simulink model "Sub1"  (R2024a)
settings: Solver=FixedStepDiscrete  StartTime=0.0  StopTime=1  FixedStep=7.5e-05  RelTol=1e-3  EnableMultiTasking=on
undefined symbols (not defined in the file or in its folder): D1, D11, Delta
libraries: spsSeriesRLCBranchLib x41, spsLoadFlowBusLib x29, spsDistributedParametersLineLib x19, spsThreePhaseSeriesRLCLoadLib x15, spsThreePhaseTransformerTwoWindingsLib x13, spsThreePhaseParallelRLCLoadLib x11, spsThreePhaseVIMeasurementLib x11, spsSynchronousMachinepuStandardLib x7, spsExcitationSystemLib x7, spsHydraulicTurbineandGovernorLib x7, spsGenericPowerSystemStabilizerLib x7, spsMultiBandPowerSystemStabilizerLib x7
(part 3 of 5)

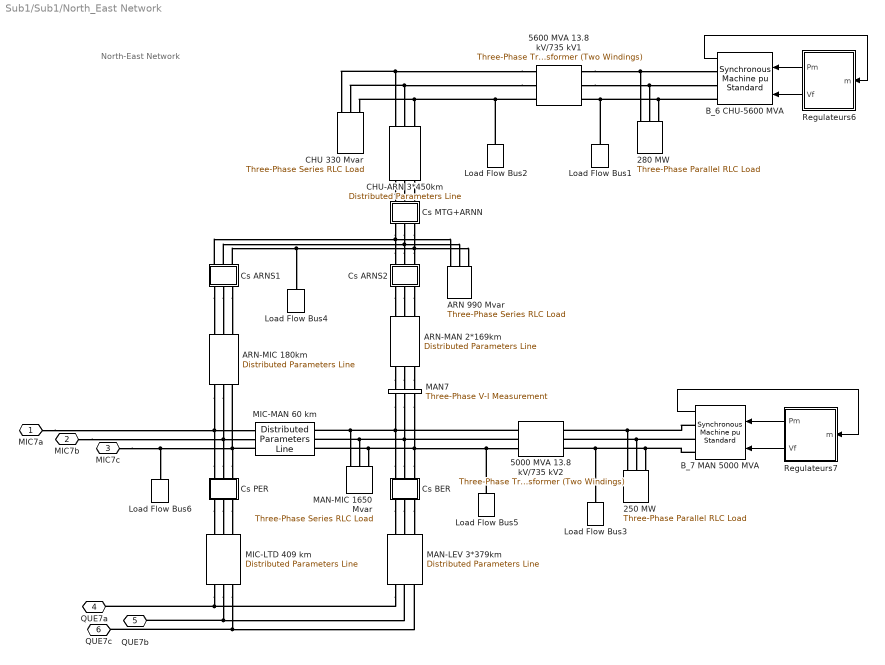
== system Sub1/Sub1/North_East Network ==
  note: North-East Network
  250 MW : spsThreePhaseParallelRLCLoadLib/Three-Phase Parallel RLC Load  LConnTagsString=A|B|C  Configuration=Y (grounded)  NominalVoltage=(13800)*1  Vabc=[1e3 1e3 1e3]  Vabcp=[1e3 1e3 1e3]  NominalFrequency=60  UnbalancedPower=off  ActivePower=250000000  InductivePower=0  CapacitivePower=0  Pabc=[10e3 9e3 11e3]  QLabc=[100 90 110]  QCabc=[100 90 110]  Pabcp=[10e3 9e3 11e3]  QLabcp=[100 90 110]  QCabcp=[100 90 110]  Measurements=None  LoadType=constant PQ
  280 MW : spsThreePhaseParallelRLCLoadLib/Three-Phase Parallel RLC Load  LConnTagsString=A|B|C  Configuration=Y (grounded)  NominalVoltage=(13800)*1  Vabc=[1e3 1e3 1e3]  Vabcp=[1e3 1e3 1e3]  NominalFrequency=60  UnbalancedPower=off  ActivePower=280000000  InductivePower=0  CapacitivePower=0  Pabc=[10e3 9e3 11e3]  QLabc=[100 90 110]  QCabc=[100 90 110]  Pabcp=[10e3 9e3 11e3]  QLabcp=[100 90 110]  QCabcp=[100 90 110]  Measurements=None  LoadType=constant PQ
  5000 MVA 13.8 kV/735 kV2 : spsThreePhaseTransformerTwoWindingsLib/Three-Phase Transformer (Two Windings)  Winding1Connection=Delta (D1)  Winding2Connection=Yg  CoreType=Three single-phase transformers  SetSaturation=off  Hysteresis=off  DataFile='basic_model'  SetInitialFlux=off  Measurements=None  UNITS=pu  NominalPower=[ 5000e6 60 ]  Winding1="[ 13.8e3 0.002  0.0]"  Winding2=[ 735e3 0.002 0.12]  Rm=500  Lm=500  L0=0.5  Saturation="[ 0,0  ;  0.005,1.2  ;  1.0,1.4 ]"  InitialFluxes=[ 0.8 , -0.8 , 0.7 ]  BreakLoop=off  DiscreteSolver=Trapezoidal iterative  DataType=off  TransfoNumber=0
  5600 MVA 13.8 kV/735 kV1 : spsThreePhaseTransformerTwoWindingsLib/Three-Phase Transformer (Two Windings)  Winding1Connection=Delta (D1)  Winding2Connection=Yg  CoreType=Three single-phase transformers  SetSaturation=off  Hysteresis=off  DataFile='basic_model'  SetInitialFlux=off  Measurements=None  UNITS=pu  NominalPower=[ 5600e6 60 ]  Winding1="[ 13.8e3 0.002  0.0]"  Winding2=[ 735e3 0.002 0.12]  Rm=500  Lm=500  L0=0.5  Saturation="[ 0,0  ;  0.005,1.2  ;  1.0,1.4 ]"  InitialFluxes=[ 0.8 , -0.8 , 0.7 ]  BreakLoop=off  DiscreteSolver=Trapezoidal iterative  DataType=off  TransfoNumber=0
  ARN 990 Mvar : spsThreePhaseSeriesRLCLoadLib/Three-Phase Series RLC Load  LConnTagsString=A|B|C  Configuration=Y (grounded)  NominalVoltage=735e3  Vabc=[1e3 1e3 1e3]  Vabcp=[1e3 1e3 1e3]  NominalFrequency=60  UnbalancedPower=off  ActivePower=3300000  InductivePower=990e6  CapacitivePower=0  Pabc=[10e3 9e3 11e3]  QLabc=[100 90 110]  QCabc=[100 90 110]  Pabcp=[10e3 9e3 11e3]  QLabcp=[100 90 110]  QCabcp=[100 90 110]  Measurements=None  LoadType=constant Z
  ARN-MAN 2*169km : spsDistributedParametersLineLib/Distributed Parameters Line  Phases=3  Length=169  Frequency=60  Resistance="[0.01273  0.3864]/2"  Inductance="[0.9337e-3  4.1264e-3]/2"  Capacitance=[12.74e-9 7.751e-9]*2  x1=[-0.000975 1.40296657323216e-09 347873.977312495 -681165.145140608;-0.0009 1.33832794722541e-09 366991.883229389 -671058.367401907;-0.000825 1.27261948233475e-09 385816.421449993 -660415.155871841;-0.00075 1.20589370490164e-09 404332.543926479 -649244.018570862;-0.000675 1.13820395449163e-09 422525.449153847 -637553.885535204;-0.0006 1.0696043412555e-09 440380.594002016 -625354.101678351;-0.000525 1.00014970267447e-09 457883.70534139 -612654.419320855;-0.00045 9.29895559723926e-10 475020.791452569 -599464.990394481;-0.000375 8.58898072490815e-10 491778.153211123 -585796.358326908;-0.0003 7.87213995280137e-10 508142.395038458 -571659.449613472;-0.000225 7.1490063124641e-10 524100.435610038 -557065.565082699;-0.00015 6.4201578658641e-10 539639.518312398 -542026.370862587;-7.5e-05 5.68617724329785e-10 554747.22144058 -526553.88905489]  x2=[-0.000975 1.15383562490741e-09 232985.418240247 -689450.364518719;-0.0009 1.12361481292558e-09 252383.458947585 -682588.200671908;-0.000825 1.09249580045418e-09 271579.748179437 -675180.38626143;-0.00075 1.06050346355564e-09 290558.940715904 -667232.84298078;-0.000675 1.02766337641458e-09 309305.864880863 -658751.923974457;-0.0006 9.940017908942e-10 327805.534669975 -649744.408759351;-0.000525 9.59545615550911e-10 346043.161730265 -640217.497805305;-0.00045 9.24322394124092e-10 364004.167181706 -630178.80677917;-0.000375 8.88360283518016e-10 381674.193271352 -619636.360456955;-0.0003 8.51688031293665e-10 399039.114850707 -608598.586308945;-0.000225 8.14334952688361e-10 416085.050667155 -597074.30776291;-0.00015 7.76330907181621e-10 432798.374460414 -585072.737150793;-7.5e-05 7.37706274625941e-10 449165.725855166 -572603.46834451]  x3=[-0.000975 -7.73577503889558e-12 1583.75858462524 -1421.24992657483;-0.0009 -7.93874680673473e-12 1623.30400424471 -1375.90902523544;-0.000825 -8.13537246184348e-12 1661.55177948056 -1329.46824327338;-0.00075 -8.3254948246816e-12 1698.4713356465 -1281.96470473921;-0.000675 -8.50896191434122e-12 1734.0331598142 -1233.43638323478;-0.0006 -8.68562707003799e-12 1768.20882440554 -1183.9220715578;-0.000525 -8.85534906834953e-12 1800.97100991715 -1133.46135069143;-0.00045 -9.01799223610721e-12 1832.29352675922 -1082.09455816387;-0.000375 -9.17342655885125e-12 1862.15133619103 -1029.8627558031;-0.0003 -9.32152778476228e-12 1890.52057033656 -976.807696912781;-0.000225 -9.46217752398633e-12 1917.37855126409 -922.971792895205;-0.00015 -9.59526334327388e-12 1942.70380911462 -868.398079348331;-7.5e-05 -9.72067885585727e-12 1966.47609926451 -813.130181663762]  x4=[-0.000975 1.24888211846857e-11 1569.30174481143 -9115.59279820371;-0.0009 1.24221857541019e-11 1826.37892658961 -9067.58416140515;-0.000825 1.23456202182921e-11 2081.99612899841 -9012.32703656664;-0.00075 1.22591857825741e-11 2335.94901555729 -8949.86559538834;-0.000675 1.21629515413134e-11 2588.03458021436 -8880.24976859062;-0.0006 1.20569944226899e-11 2838.05130962626 -8803.53520600026;-0.000525 1.19413991272031e-11 3085.79934424489 -8719.78323206483;-0.00045 1.18162580599636e-11 3331.08063808204 -8629.06079683085;-0.000375 1.16816712568257e-11 3573.69911702436 -8531.44042242494;-0.0003 1.15377463044207e-11 3813.46083557195 -8427.00014508076;-0.000225 1.13845982541534e-11 4050.17413187549 -8315.82345275802;-0.00015 1.12223495302319e-11 4283.64978094776 -8197.99921840352;-7.5e-05 1.10511298318037e-11 4513.70114592717 -8073.62162890742]  x5=0.000955765248222805  V1=ones(3,3)  V2=ones(3,3)  I1=ones(3,3)  I2=ones(3,3)  nHarmo=1  Measurements=None  Decoupling=on  VsMag0=[624500.542746134 624501.904306159 624500.043261812]  VrMag0=[594207.380493459 594208.101305642 594207.286862208]  VsAngle0=[18.1135948354262 -101.886530201493 138.113424134256]  VrAngle0=[9.73160889880125 -110.268441654035 129.731523430557]  IsMag0=[1744.35611857435 1744.39210598318 1744.37536737656]  IrMag0=[7582.44376493559 7582.43378992651 7582.40838116995]  IsAngle0=[39.1559168024892 -80.8440356055455 159.154916919477]  IrAngle0=[0.828149284036614 -119.172115933988 120.828081951992]
      settings: AttributesFormatString=\n  LibrarySourceBlock=sps_lib/Power Grid Elements/Distributed Parameters Line
  ARN-MIC 180km : spsDistributedParametersLineLib/Distributed Parameters Line  Phases=3  Length=180  Frequency=60  Resistance="[0.01273  0.3864]"  Inductance="[0.9337e-3  4.1264e-3]"  Capacitance=[12.74e-9 7.751e-9]  x1=[-0.00105 1.26488530745679e-09 336203.730988093 -674396.627297763;-0.000975 1.2044174612995e-09 355134.952563311 -664622.476598035;-0.0009 1.14298682225185e-09 373782.284691197 -654317.03685958;-0.000825 1.08064249702677e-09 392130.820979761 -643488.546093246;-0.00075 1.01743432272396e-09 410165.893889837 -632145.660428869;-0.000675 9.53412826990829e-10 427873.086460087 -620297.447195699;-0.0006 8.88629187631506e-10 445238.243831697 -607953.377674109;-0.000525 8.23135191696074e-10 462247.484563562 -595123.319524406;-0.00045 7.5698319408279e-10 478887.211728891 -581817.528898766;-0.000375 6.90226075686387e-10 495144.123784384 -568046.642242632;-0.0003 6.22917201125894e-10 511005.225203283 -553821.667792094;-0.000225 5.55110376085774e-10 526457.836863796 -539153.976774079;-0.00015 4.86859804304484e-10 541489.606184596 -524055.294316363;-7.5e-05 4.18220044244838e-10 556088.51699928 -508537.690074686]  x2=[-0.00105 4.67164063168132e-09 192165.578486796 -719334.039084833;-0.000975 4.62687418731474e-09 212424.764832653 -713613.931123211;-0.0009 4.57840909051637e-09 232514.142071711 -707323.371103708;-0.000825 4.52628408354304e-09 252417.651063182 -700467.387603755;-0.00075 4.47054083432781e-09 272119.381246513 -693051.461191662;-0.000675 4.41122390317118e-09 291603.583360041 -685081.520045535;-0.0006 4.34838070712034e-09 310854.682030716 -676563.935214383;-0.000525 4.28206148206469e-09 329857.288224812 -667505.515525196;-0.00045 4.21231924257801e-09 348596.211549686 -657913.502140075;-0.000375 4.13920973953947e-09 367056.472396749 -647795.562767757;-0.0003 4.06279141556716e-09 385223.31391593 -637159.785534167;-0.000225 3.98312535830005e-09 403082.213812081 -626014.672516893;-0.00015 3.90027525156537e-09 420618.895953875 -614369.132948754;-7.5e-05 3.8143073244708e-09 437819.341785928 -602232.476095899]  x3=[-0.00105 2.81387396252104e-12 149.00166074934 -364.54093553834;-0.000975 3.09923380082505e-12 159.247423691766 -360.183291872447;-0.0009 3.38211615904855e-12 169.36588668026 -355.53772319402;-0.000825 3.66229490536262e-12 179.348961170327 -350.607943099582;-0.00075 3.93954606916433e-12 189.188666844966 -345.397892379912;-0.000675 4.21364802011543e-12 198.877137994012 -339.911735869838;-0.0006 4.48438164531022e-12 208.406629801869 -334.153859118933;-0.000525 4.7515305244311e-12 217.76952453859 -328.128864885774;-0.00045 5.0148811027516e-12 226.95833764938 -321.841569458566;-0.000375 5.27422286184881e-12 235.965723737633 -315.296998805074;-0.0003 5.52934848788858e-12 244.784482436726 -308.500384554942;-0.000225 5.780054037349e-12 253.407564165887 -301.457159817612;-0.00015 6.02613910004975e-12 261.82807576552 -294.172954839173;-7.5e-05 6.26740695935695e-12 270.03928600749 -286.653592501632]  x4=[-0.00105 5.46621407801285e-12 1187.65933351911 -4979.4651542706;-0.000975 5.11013850401405e-12 1327.95758028632 -4943.89904376687;-0.0009 4.74997796348289e-12 1467.19427808228 -4904.38085601174;-0.000825 4.38602036324481e-12 1605.25812322116 -4860.94218123987;-0.00075 4.01855664543673e-12 1742.03874957762 -4813.61774366322;-0.000675 3.64788055493226e-12 1877.42681681175 -4762.44537371311;-0.0006 3.27428840452662e-12 2011.31409777411 -4707.46597779911;-0.000525 2.89807883806869e-12 2143.59356502085 -4648.7235056091;-0.00045 2.5195525917297e-12 2274.1594763698 -4586.26491497656;-0.000375 2.13901225359934e-12 2402.90745942914 -4520.1401343432;-0.0003 1.75676202180143e-12 2529.73459503113 -4450.40202284691;-0.000225 1.37310746132265e-12 2654.53949950409 -4377.10632806698;-0.00015 9.88355259748543e-13 2777.22240571696 -4300.31164146037;-7.5e-05 6.02812982102133e-13 2897.68524283163 -4220.07935152456]  x5=0.00101797482059234  V1=ones(3,3)  V2=ones(3,3)  I1=ones(3,3)  I2=ones(3,3)  nHarmo=1  Measurements=None  Decoupling=on  VsMag0=[615273.936100305 615275.237958967 615273.425866952]  VrMag0=[607930.231676096 607930.976808471 607930.152146782]  VsAngle0=[19.177410374195 -100.822714483797 139.17724295489]  VrAngle0=[7.63692875075284 -112.363120449628 127.636843332424]  IsMag0=[322.89615060232 322.910343515199 322.909058921661]  IrMag0=[4197.50413399089 4197.49907033583 4197.48826872769]  IsAngle0=[14.9112658694594 -105.087543385527 134.909680310757]  IrAngle0=[6.09512812442934 -113.905082032176 126.095082904974]
      settings: AttributesFormatString=\n  LibrarySourceBlock=sps_lib/Power Grid Elements/Distributed Parameters Line
  "B_6 CHU-5600 MVA " : spsSynchronousMachinepuStandardLib/Synchronous Machine pu Standard  PresetModel=No  MechanicalLoad=Mechanical power Pm  ShowDetailedParameters=on  RotorType=Salient-pole  Units=per unit standard parameters  MeasurementBus=off  NominalParameters="[ 5600E6  13800   60 ]"  Reactances1=[ 31 32 33 34 35 36 37 ]  Reactances2=[ 1.305, 0.296, 0.252, 0.474, 0.243, 0.18 ]  dAxisTimeConstants=Short-circuit  qAxisTimeConstants=Open-circuit  TimeConstants1=[]  TimeConstants2=[]  TimeConstants3=[]  TimeConstants4=[]  TimeConstants5=[ 1.01, 0.053, 0.1 ]  TimeConstants6=[]  TimeConstants7=[]  TimeConstants8=[]  StatorResistance=2.8544e-3  Mechanical="[ 4.0 0  32]"  PolePairs=32  InitialConditions=[0 -61.7964 0.894782 0.894782 0.894782 8.48442 -111.516 128.484 1.31361]  SetSaturation=off  Saturation=[0.6404,0.7127,0.8441,0.9214,0.9956,1.082,1.19,1.316,1.457;0.7,0.7698,0.8872,0.9466,0.9969,1.046,1.1,1.151,1.201]  LoadFlowParameters=[1 5000000000 0 0 0]  TsPowergui=0  TsBlock=-1  IterativeModel=Trapezoidal non iterative  IterativeDiscreteModel=Trapezoidal non iterative  BusType=PV  Pref=5000000000  Qref=0  Qmin=-Inf  Qmax=Inf  PLF=0  QLF=0
  B_7 MAN 5000 MVA : spsSynchronousMachinepuStandardLib/Synchronous Machine pu Standard  PresetModel=No  MechanicalLoad=Mechanical power Pm  ShowDetailedParameters=on  RotorType=Salient-pole  Units=per unit standard parameters  MeasurementBus=off  NominalParameters="[ 5000E6  13800   60 ]"  Reactances1=[ 31 32 33 34 35 36 37 ]  Reactances2=[ 1.305, 0.296, 0.252, 0.474, 0.243, 0.18 ]  dAxisTimeConstants=Short-circuit  qAxisTimeConstants=Open-circuit  TimeConstants1=[]  TimeConstants2=[]  TimeConstants3=[]  TimeConstants4=[]  TimeConstants5=[ 1.01, 0.053, 0.1 ]  TimeConstants6=[]  TimeConstants7=[]  TimeConstants8=[]  StatorResistance=2.8544e-3  Mechanical="[ 3.7 0  32]"  PolePairs=32  InitialConditions=[0 -81.9543 0.907703 0.907703 0.907703 -8.76021 -128.76 111.24 1.25655]  SetSaturation=off  Saturation=[0.6404,0.7127,0.8441,0.9214,0.9956,1.082,1.19,1.316,1.457;0.7,0.7698,0.8872,0.9466,0.9969,1.046,1.1,1.151,1.201]  LoadFlowParameters=[1 4500000000 0 0 0]  TsPowergui=0  TsBlock=-1  IterativeModel=Trapezoidal non iterative  IterativeDiscreteModel=Trapezoidal non iterative  BusType=PV  Pref=4500000000  Qref=0  Qmin=-Inf  Qmax=Inf  PLF=0  QLF=0
  CHU 330 Mvar : spsThreePhaseSeriesRLCLoadLib/Three-Phase Series RLC Load  LConnTagsString=A|B|C  Configuration=Y (grounded)  NominalVoltage=735e3  Vabc=[1e3 1e3 1e3]  Vabcp=[1e3 1e3 1e3]  NominalFrequency=60  UnbalancedPower=off  ActivePower=1100000  InductivePower=330e6  CapacitivePower=0  Pabc=[10e3 9e3 11e3]  QLabc=[100 90 110]  QCabc=[100 90 110]  Pabcp=[10e3 9e3 11e3]  QLabcp=[100 90 110]  QCabcp=[100 90 110]  Measurements=None  LoadType=constant Z
  CHU-ARN 3*450km : spsDistributedParametersLineLib/Distributed Parameters Line  Phases=3  Length=450  Frequency=60  Resistance="[0.01273  0.3864]/3"  Inductance="[0.9337e-3  4.1264e-3]/3"  Capacitance=[12.74e-9 7.751e-9]*3  x1=[-0.00255 2.06397121919185e-09 0 0;-0.002475 1.97424505917164e-09 0 0;-0.0024 1.88294071785809e-09 0 0;-0.002325 1.79013118254465e-09 0 0;-0.00225 1.6958906437538e-09 0 0;-0.002175 1.60029443593034e-09 0 0;-0.0021 1.50341897722012e-09 0 0;-0.002025 1.40534170838259e-09 0 0;-0.00195 1.30614103088583e-09 0 0;-0.001875 1.20589624423361e-09 0 0;-0.0018 1.10468748257457e-09 0 0;-0.001725 1.00259565064426e-09 0 0;-0.00165 8.99702359091042e-10 0 0;-0.001575 7.96089859237878e-10 336692.1296535 -649852.524072587;-0.0015 6.91840977331823e-10 354929.318551946 -640074.408280256;-0.001425 5.8703904833401e-10 372882.782383741 -629784.626799413;-0.00135 4.81767849302958e-10 390538.169424598 -618991.405123934;-0.001275 3.76111532424469e-10 407881.36622825 -607703.371190085;-0.0012 2.70154557741658e-10 424898.508908534 -595929.54847948;-0.001125 1.63981625638893e-10 441575.994221962 -583679.348805849;-0.00105 5.76776091335941e-11 457900.490441947 -570962.564791376;-0.000975 -4.86725139699487e-11 473858.948015986 -557789.362038628;-0.0009 -1.54983729010538e-10 489438.609997266 -544170.271004331;-0.000825 -2.61171052429488e-10 504627.022242376 -530116.178581477;-0.00075 -3.67149599705176e-10 519412.043366958 -515638.319396514;-0.000675 -4.72834653208437e-10 533781.854451343 -500748.266828557;-0.0006 -5.78141729924536e-10 547724.968488416 -485457.923757802;-0.000525 -6.82986648987598e-10 561230.239566152 -469779.513050551;-0.00045 -7.87285598973506e-10 574286.87177749 -453725.567788435;-0.000375 -8.90955204897468e-10 586884.427850413 -437308.921249662;-0.0003 -9.93912594862707e-10 599012.837491345 -420542.696650294;-0.000225 -1.09607546630699e-09 610662.40543519 -403440.296653742;-0.00015 -1.19736215179401e-09 621823.819195578 -386015.392656889;-7.5e-05 -1.29769168429716e-09 632488.156509125 -368281.913861379]  x2=[-0.00255 2.57099365854968e-09 0 0;-0.002475 2.5533409835626e-09 0 0;-0.0024 2.53364720686069e-09 0 0;-0.002325 2.51192807134772e-09 0 0;-0.00225 2.4882009389683e-09 0 0;-0.002175 2.46248477682902e-09 0 0;-0.0021 2.43480014203643e-09 0 0;-0.002025 2.40516916526398e-09 0 0;-0.00195 2.37361553306114e-09 0 0;-0.001875 2.34016446891871e-09 0 0;-0.0018 2.30484271310554e-09 0 0;-0.001725 2.26767850129279e-09 0 0;-0.00165 2.22870154198275e-09 0 0;-0.001575 2.18794299276033e-09 24661.218637955 -733238.39673676;-0.0015 2.14543543538615e-09 45380.4401577776 -732248.159297617;-0.001425 2.10121284975118e-09 66063.3852480821 -730672.573883705;-0.00135 2.05531058671375e-09 86693.520279023 -728512.899993896;-0.001275 2.00776533984062e-09 107254.353836308 -725770.864038452;-0.0012 1.95861511607465e-09 127729.449904183 -722448.657958963;-0.001125 1.90789920535271e-09 148102.441004131 -718548.937476136;-0.00105 1.85565814919785e-09 168357.041278783 -714074.819966858;-0.000975 1.80193370831104e-09 188477.059510587 -709029.881972211;-0.0009 1.74676882918832e-09 208446.412064813 -703418.156338435;-0.000825 1.69020760979e-09 228249.135746572 -697244.128993141;-0.00075 1.63229526428946e-09 247869.400561543 -690512.735359323;-0.000675 1.5730780869296e-09 267291.522370235 -683229.356410058;-0.0006 1.51260341501596e-09 286499.975425642 -675399.814367038;-0.000525 1.45091959107596e-09 305479.40478429 -667030.368046378;-0.00045 1.38807592421466e-09 324214.638580745 -658127.707855407;-0.000375 1.32412265069782e-09 342690.700155768 -648698.950444469;-0.0003 1.25911089379378e-09 360892.820028431 -638751.633017972;-0.000225 1.19309262290627e-09 378806.447702609 -628293.707309268;-0.00015 1.12612061203094e-09 396417.263298426 -617333.533224158;-7.5e-05 1.05824839756858e-09 413711.188999349 -605879.872158107]  x3=[-0.00255 1.88883345001377e-12 0 0;-0.002475 1.79513657119373e-12 0 0;-0.0024 1.70000468766518e-12 0 0;-0.002325 1.60351384640027e-12 0 0;-0.00225 1.50574118070112e-12 0 0;-0.002175 1.40676484854074e-12 0 0;-0.0021 1.30666397008465e-12 0 0;-0.002025 1.20551856444351e-12 0 0;-0.00195 1.10340948570701e-12 0 0;-0.001875 1.00041835831036e-12 0 0;-0.0018 8.96627511784997e-13 0 0;-0.001725 7.92119914945571e-13 0 0;-0.00165 6.86979109565978e-13 0 0;-0.001575 5.81289143597332e-13 -336.540930618725 -2064.60581280642;-0.0015 4.75134503981316e-13 -278.039507495945 -2073.29664773679;-0.001425 3.68600049112618e-13 -219.31582384502 -2080.33012104946;-0.00135 2.6177094100443e-13 -160.416822480158 -2085.70061029348;-0.001275 1.54732577211233e-13 -101.389586361865 -2089.40382238193;-0.0012 4.75705225633011e-14 -42.281300959547 -2091.43679702371;-0.001125 -5.96295592325144e-14 16.8607834678324 -2091.79790909;-0.00105 -1.66781974071043e-13 75.9893896428864 -2090.48686991336;-0.000975 -2.73801065951348e-13 135.057251062536 -2087.50472751842;-0.0009 -3.80601285448829e-13 194.017149782132 -2082.8538657842;-0.000825 -4.87097258102117e-13 252.821954160754 -2076.5380025384;-0.00075 -5.93203852660115e-13 311.424656537526 -2068.56218658548;-0.000675 -6.98836249134622e-13 369.778410808818 -2058.93279367065;-0.0006 -8.03910006604122e-13 427.83656987631 -2047.6575213833;-0.000525 -9.08341130714579e-13 485.552722935961 -2034.74538300356;-0.00045 -1.01204614082323e-12 542.880732578103 -2020.2067002973;-0.000375 -1.11494213673173e-12 599.774771668976 -2004.05309526502;-0.0003 -1.21694686495531e-12 656.189359984238 -1986.29748085143;-0.000225 -1.31797878447496e-12 712.079400565163 -1966.95405062301;-0.00015 -1.41795713192005e-12 767.400215768456 -1946.03826742193;-7.5e-05 -1.51680198612936e-12 822.107582980881 -1923.56685100526]  x4=[-0.00255 1.87200405385975e-11 0 0;-0.002475 1.85935736833939e-11 0 0;-0.0024 1.84522434098792e-11 0 0;-0.002325 1.82961626953113e-11 0 0;-0.00225 1.81254563082255e-11 0 0;-0.002175 1.79402607086956e-11 0 0;-0.0021 1.77407239392505e-11 0 0;-0.002025 1.75270055065304e-11 0 0;-0.00195 1.72992762537807e-11 0 0;-0.001875 1.70577182242814e-11 0 0;-0.0018 1.68025245158255e-11 0 0;-0.001725 1.6533899126359e-11 0 0;-0.00165 1.62520567909079e-11 0 0;-0.001575 1.5957222809923e-11 -291.743024305016 -14207.2379327602;-0.0015 1.56496328691775e-11 110.022151991571 -14209.8063832445;-0.001425 1.53295328513638e-11 511.699378263252 -14201.0157319234;-0.00135 1.49971786395385e-11 912.967559881212 -14180.8730059089;-0.001275 1.46528359125732e-11 1313.50592920067 -14149.3943069882;-0.0012 1.42967799327754e-11 1712.99430197765 -14106.6047987515;-0.001125 1.39292953258473e-11 2111.11333331931 -14052.5386864769;-0.00105 1.35506758533612e-11 2507.54477296344 -13987.2391897874;-0.000975 1.31612241779301e-11 2901.97171968278 -13910.7585081016;-0.0009 1.27612516212647e-11 3294.07887461107 -13823.1577789061;-0.000825 1.23510779153069e-11 3683.55279328808 -13724.5070288835;-0.00075 1.19310309466415e-11 4070.08213622239 -13614.8851179341;-0.000675 1.15014464943883e-11 4453.35791777135 -13494.3796761361;-0.0006 1.10626679617854e-11 4833.0737531395 -13363.0870336959;-0.000525 1.06150461016784e-11 5208.9261032979 -13221.1121439431;-0.00045 1.01589387361334e-11 5580.61451762857 -13068.5684994323;-0.000375 9.69471047039966e-12 5947.84187410011 -12905.5780412187;-0.0003 9.22273240144994e-12 6310.31461678253 -12732.271061381;-0.000225 8.74338182133104e-12 6667.74299051134 -12548.7860988672;-0.00015 8.2570419155624e-12 7019.84127251342 -12355.2698287487;-7.5e-05 7.76410145682344e-12 7366.32800080944 -12151.8769449711]  x5=0.00254493705148084  V1=ones(3,3)  V2=ones(3,3)  I1=ones(3,3)  I2=ones(3,3)  nHarmo=1  Measurements=None  Decoupling=on  VsMag0=[597589.636778609 597591.191030852 597588.179734018]  VrMag0=[599025.218159228 599025.68105058 599025.14641922]  VsAngle0=[31.4089201475996 -88.5913271983242 151.408667420091]  VrAngle0=[5.94632207994603 -114.053711405461 125.946266994132]  IsMag0=[1726.12548309445 1726.1686602899 1726.16794416464]  IrMag0=[11726.0675753704 11726.049206286 11726.0164561745]  IsAngle0=[-5.2389877444989 -125.238187761882 114.760171100741]  IrAngle0=[2.84375678806612 -117.156479810911 122.843716218958]
      settings: AttributesFormatString=\n  LibrarySourceBlock=sps_lib/Power Grid Elements/Distributed Parameters Line
  "Cs ARNS1 " : Subsystem  mask{Xc=25}
      mask prompts: Xc "Condensator Reactance at  60Hz  (ohm):"
      mask help: Series Compensation
      mask init:
      | Cs=1/Xc/(2*pi*60);
      mask Display: disp('Cs')
  Cs ARNS2 : Subsystem  mask{Xc=25/2}
      mask prompts: Xc "Condensator Reactance at  60Hz  (ohm):"
      mask help: Series Compensation
      mask init:
      | Cs=1/Xc/(2*pi*60);
      mask Display: disp('Cs')
  Cs BER : Subsystem  mask{Xc=22/3}
      mask prompts: Xc "Condensator Reactance at  60Hz  (ohm):"
      mask help: Series Compensation
      mask init:
      | Cs=1/Xc/(2*pi*60);
      mask Display: disp('Cs')
  "Cs MTG+ARNN " : Subsystem  mask{Xc=(30+25)/3}
      mask prompts: Xc "Condensator Reactance at  60Hz  (ohm):"
      mask help: Series Compensation
      mask init:
      | Cs=1/Xc/(2*pi*60);
      mask Display: disp('Cs')
  "Cs PER " : Subsystem  mask{Xc=22}
      mask prompts: Xc "Condensator Reactance at  60Hz  (ohm):"
      mask help: Series Compensation
      mask init:
      | Cs=1/Xc/(2*pi*60);
      mask Display: disp('Cs')
  Load Flow Bus1 : spsLoadFlowBusLib/Load Flow Bus  LConnTagsString=a  Phases=single  Connectors=on one side  ID=CHU_13.8  Vbase=13.8e3  Vref=1  Vangle=0  VLF=1  VLFb=1  VLFc=1  angleLF=4.726  angleLFb=0  angleLFc=0
      settings: AttributesFormatString=%<ID>\n%<Vbase>V\n%<VLF>pu\n%<angleLF>deg.
  Load Flow Bus2 : spsLoadFlowBusLib/Load Flow Bus  LConnTagsString=a  Phases=single  Connectors=on one side  ID=CHU7  Vbase=735e3  Vref=1  Vangle=0  VLF=1.009  VLFb=1  VLFc=1  angleLF=28.97  angleLFb=0  angleLFc=0
      settings: AttributesFormatString=%<ID>\n%<Vbase>V\n%<VLF>pu\n%<angleLF>deg.
  Load Flow Bus3 : spsLoadFlowBusLib/Load Flow Bus  LConnTagsString=a  Phases=single  Connectors=on one side  ID=MAN_13.8  Vbase=13.8e3  Vref=1  Vangle=0  VLF=1  VLFb=1  VLFc=1  angleLF=-16.23  angleLFb=0  angleLFc=0
      settings: AttributesFormatString=%<ID>\n%<Vbase>V\n%<VLF>pu\n%<angleLF>deg.
  Load Flow Bus4 : spsLoadFlowBusLib/Load Flow Bus  LConnTagsString=a  Phases=single  Connectors=on one side  ID=ARN7  Vbase=735e3  Vref=1  Vangle=0  VLF=1.054  VLFb=1  VLFc=1  angleLF=12.72  angleLFb=0  angleLFc=0
      settings: AttributesFormatString=%<ID>\n%<Vbase>V\n%<VLF>pu\n%<angleLF>deg.
  Load Flow Bus5 : spsLoadFlowBusLib/Load Flow Bus  LConnTagsString=a  Phases=single  Connectors=on one side  ID=MAN7  Vbase=735e3  Vref=1  Vangle=0  VLF=1.016  VLFb=1  VLFc=1  angleLF=7.996  angleLFb=0  angleLFc=0
      settings: AttributesFormatString=%<ID>\n%<Vbase>V\n%<VLF>pu\n%<angleLF>deg.
  Load Flow Bus6 : spsLoadFlowBusLib/Load Flow Bus  LConnTagsString=a  Phases=single  Connectors=on one side  ID=MIC7  Vbase=735e3  Vref=1  Vangle=0  VLF=1.041  VLFb=1  VLFc=1  angleLF=5.981  angleLFb=0  angleLFc=0
      settings: AttributesFormatString=%<ID>\n%<Vbase>V\n%<VLF>pu\n%<angleLF>deg.
  MAN-LEV 3*379km : spsDistributedParametersLineLib/Distributed Parameters Line  Phases=3  Length=379  Frequency=60  Resistance="[0.01273  0.3864]/3"  Inductance="[0.9337e-3  4.1264e-3]/3"  Capacitance=[12.74e-9 7.751e-9]*3  x1=[-0.002175 2.70792225183745e-09 -30838.3336726704 -721772.968423957;-0.0021 2.6646615578597e-09 -10421.0500053613 -722356.328523207;-0.002025 2.61927077420328e-09 10004.5640898749 -722362.248025858;-0.00195 2.57178618556614e-09 30422.1806896527 -721790.722199949;-0.001875 2.52224575040192e-09 50815.478263662 -720642.207914483;-0.0018 2.47068907057647e-09 71168.1547218502 -718917.623274205;-0.001725 2.41715735971082e-09 91463.9404460632 -716618.34688569;-0.00165 2.36169341023557e-09 111686.611295729 -713746.216755303;-0.001575 2.30434155918329e-09 131820.001577187 -710303.528819926;-0.0015 2.24514765274621e-09 151848.016966298 -706293.035111618;-0.001425 2.18415900962743e-09 171754.647373999 -701717.941557688;-0.00135 2.12142438321512e-09 191523.979744523 -696581.905417921;-0.001275 2.05699392260974e-09 211140.210776055 -690889.032361023;-0.0012 1.99091913253569e-09 230587.659553645 -684643.873182613;-0.001125 1.92325283216917e-09 249850.780084298 -677851.420167383;-0.00105 1.85404911291538e-09 268914.173724197 -670517.103098346;-0.000975 1.78336329516862e-09 287762.601488146 -662646.784916348;-0.0009 1.71125188409008e-09 306380.99623138 -654246.757033323;-0.000825 1.63777252443842e-09 324754.474694014 -645323.734303037;-0.00075 1.5629839544895e-09 342868.349398487 -635884.849653334;-0.000675 1.48694595908181e-09 360708.140390512 -625937.648384182;-0.0006 1.40971932182546e-09 378259.586814129 -615490.082136079;-0.000525 1.33136577651268e-09 395508.658311613 -604550.50253363;-0.00045 1.25194795776873e-09 412441.566239128 -593127.654509389;-0.000375 1.17152935098279e-09 429044.774689159 -581230.669313291;-0.0003 1.09017424155867e-09 445305.011310908 -568869.05721327;-0.000225 1.00794766352608e-09 461209.277920011 -556052.699892903;-0.00015 9.24915347553379e-10 476744.860889083 -542791.842552132;-7.5e-05 8.41143668403523e-10 491899.341310801 -529097.085717419]  x2=[-0.002175 1.35798481191488e-08 -379192.175232149 -624794.196144237;-0.0021 1.36505639706313e-08 -361377.320734424 -635264.451513471;-0.002025 1.37103677701362e-08 -343273.586735762 -645226.886200037;-0.00195 1.37592117114214e-08 -324895.445084125 -654673.536386076;-0.001875 1.37970567493875e-08 -306257.586984756 -663596.85056397;-0.0018 1.38238726312902e-08 -287374.911256249 -671989.695572895;-0.001725 1.38396379209237e-08 -268262.512420667 -679845.362300967;-0.00165 1.38443400157569e-08 -248935.66863721 -687157.571048398;-0.001575 1.38379751570069e-08 -229409.829489088 -693920.476547396;-0.0015 1.38205484326445e-08 -209700.603633361 -700128.672634782;-0.001425 1.37920737733266e-08 -189823.746323616 -705777.196573591;-0.00135 1.37525739412601e-08 -169795.146815461 -710861.533020212;-0.001275 1.37020805120064e-08 -149630.815664894 -715377.617633884;-0.0012 1.36406338492402e-08 -129346.871929713 -719321.840325663;-0.001125 1.35682830724837e-08 -108959.530284185 -722691.048144279;-0.00105 1.34850860178407e-08 -88485.088057284 -725482.547796553;-0.000975 1.33911091917638e-08 -67939.9122048577 -727694.107800373;-0.0009 1.32864277178898e-08 -47340.4262261302 -729323.960268511;-0.000825 1.31711252769873e-08 -26703.0970350105 -730370.802321841;-0.00075 1.30452940400633e-08 -6044.42179669201 -730833.797130843;-0.000675 1.29090345946834e-08 14619.085259928 -730712.57458455;-0.0006 1.27624558645634e-08 35270.9060434707 -730007.231586412;-0.000525 1.26056750224974e-08 55894.5318043853 -728718.33197683;-0.00045 1.24388173966917e-08 76473.4763317904 -726846.906082429;-0.000375 1.22620163705793e-08 96991.2891322993 -724394.449892436;-0.0003 1.20754132761955e-08 117431.568580292 -721362.923862806;-0.000225 1.18791572811987e-08 137777.975029126 -717754.751349063;-0.00015 1.16734052696285e-08 158014.243872794 -713572.816669108;-7.5e-05 1.14583217164948e-08 178124.19854761 -708820.462797537]  x3=[-0.002175 3.68878771544443e-12 -359.273937221545 349.814819582881;-0.0021 5.23491407682341e-12 -369.020063583937 339.517457529602;-0.002025 6.77685572798626e-12 -378.471200953696 328.948690415565;-0.00195 8.31338006436952e-12 -387.619794236217 318.116966751493;-0.001875 9.8432588119283e-12 -396.458530186007 307.030945251554;-0.0018 1.13652690089997e-11 -404.980343252785 295.699487911711;-0.001725 1.28781939839198e-11 -413.178421229574 284.131652925585;-0.00165 1.43808243276121e-11 -421.046210698274 272.336687443471;-0.001575 1.5871958860371e-11 -428.577422268365 260.324020180305;-0.0015 1.73504055920659e-11 -435.766035604549 248.103253878499;-0.001425 1.88149826750007e-11 -442.606304239314 235.684157631649;-0.00135 2.02645193486639e-11 -449.092760166574 223.076659075277;-0.001275 2.16978568756174e-11 -455.220218212707 210.290836450827;-0.0012 2.31138494677729e-11 -460.983780181503 197.336910549276;-0.001125 2.45113652023175e-11 -466.378838769711 184.225236540789;-0.00105 2.58892869265559e-11 -471.401081250041 170.966295696951;-0.000975 2.72465131509446e-11 -476.046492918699 157.570687012205;-0.0009 2.85819589296061e-11 -480.311360304673 144.049118731174;-0.000825 2.98945567276178e-11 -484.19227413823 130.412399788654;-0.00075 3.11832572743836e-11 -487.686132076231 116.67143116912;-0.000675 3.2447030402404e-11 -490.790141182098 102.837197192643;-0.0006 3.3684865870777e-11 -493.501820158445 88.920756734191;-0.000525 3.48957741727686e-11 -495.819001330589 74.9332343833393;-0.00045 3.60787873268098e-11 -497.739832379354 60.8858115514385;-0.000375 3.72329596502858e-11 -499.26277782179 46.7897175333676;-0.0003 3.83573685155008e-11 -500.386620238611 32.6562205310072;-0.000225 3.9451115087212e-11 -501.110461247386 18.4966186456112;-0.00015 4.05133250411447e-11 -501.433722220687 4.32223084627774;-7.5e-05 4.15431492629142e-11 -501.356144748638 -9.85561207826192]  x4=[-0.002175 5.12577301080103e-11 -7842.63207577963 -13937.1348474405;-0.0021 5.04893439187957e-11 -7445.48599612264 -14153.2795346851;-0.002025 4.96805973205653e-11 -7042.3881088801 -14358.1103068222;-0.00195 4.88321368129755e-11 -6633.66064433547 -14551.4634252665;-0.001875 4.79446406423741e-11 -6219.63033297018 -14733.1843264935;-0.0018 4.70188182596208e-11 -5800.62814428025 -14903.1277455951;-0.001725 4.60554097529629e-11 -5376.98902220436 -15061.1578324024;-0.00165 4.50551852564198e-11 -4949.05161737481 -15207.148260082;-0.001575 4.40189443341501e-11 -4517.15801640536 -15340.9823261196;-0.0015 4.29475153412922e-11 -4081.65346843244 -15462.5530456106;-0.001425 4.18417547617895e-11 -3642.88610912824 -15571.7632367819;-0.00135 4.07025465237305e-11 -3201.20668240643 -15668.5255986777;-0.001275 3.95308012927503e-11 -2756.96826004281 -15752.7627809464;-0.0012 3.83274557440582e-11 -2310.52595943514 -15824.4074456734;-0.001125 3.70934718136741e-11 -1862.23665972773 -15883.4023212099;-0.00105 3.58298359294712e-11 -1412.45871652771 -15929.700247955;-0.000975 3.45375582226412e-11 -961.551675441045 -15963.2642160544;-0.0009 3.32176717202104e-11 -509.875984657262 -15984.0673949857;-0.000825 3.18712315192538e-11 -57.7927068127101 -15992.0931550059;-0.00075 3.0499313943467e-11 394.33676963741 -15987.3350804451;-0.000675 2.91030156827689e-11 846.151019307439 -15969.7969748355;-0.0006 2.76834529166251e-11 1297.28886879918 -15939.4928578704;-0.000525 2.62417604217908e-11 1747.38968541838 -15896.446954197;-0.00045 2.47790906651877e-11 2196.09366545902 -15840.6936740523;-0.000375 2.32966128826396e-11 2643.04212182485 -15772.2775857552;-0.0003 2.17955121442033e-11 3087.8777707584 -15691.2533800801;-0.000225 2.02769884068414e-11 3530.24501744812 -15597.6858265371;-0.00015 1.87422555551954e-11 3969.79024028544 -15491.649721597;-7.5e-05 1.71925404312247e-11 4406.16207354451 -15373.2298288996]  x5=0.00214340253891386  V1=ones(3,3)  V2=ones(3,3)  I1=ones(3,3)  I2=ones(3,3)  nHarmo=1  Measurements=None  Decoupling=on  VsMag0=[589863.022608851 589863.802580034 589862.857708977]  VrMag0=[596743.7373363 596743.911083318 596743.706580261]  VsAngle0=[14.533491944612 -105.46657029174 134.533395214794]  VrAngle0=[-14.2738568821649 -134.273869923457 105.726122150019]  IsMag0=[413.109398328733 413.092934232236 413.107596304831]  IrMag0=[13174.467520531 13174.4678533381 13174.4493337429]  IsAngle0=[-117.256344753939 122.744684998192 2.74614766421398]  IrAngle0=[-12.3870102586405 -132.387102424574 107.612942404924]
      settings: AttributesFormatString=\n  LibrarySourceBlock=sps_lib/Power Grid Elements/Distributed Parameters Line
  MAN-MIC 1650 Mvar : spsThreePhaseSeriesRLCLoadLib/Three-Phase Series RLC Load  LConnTagsString=A|B|C  Configuration=Y (grounded)  NominalVoltage=735e3  Vabc=[1e3 1e3 1e3]  Vabcp=[1e3 1e3 1e3]  NominalFrequency=60  UnbalancedPower=off  ActivePower=5500000  InductivePower=1650e6  CapacitivePower=0  Pabc=[10e3 9e3 11e3]  QLabc=[100 90 110]  QCabc=[100 90 110]  Pabcp=[10e3 9e3 11e3]  QLabcp=[100 90 110]  QCabcp=[100 90 110]  Measurements=None  LoadType=constant Z
  MAN7 : spsThreePhaseVIMeasurementLib/Three-Phase V-I Measurement  VoltageMeasurement=no  SetLabelV=on  LabelV=Vabc_MAN7  Vpu=on  VpuLL=off  CurrentMeasurement=no  SetLabelI=on  LabelI=Iabc_MAN7  Ipu=on  Pbase=100e6  Vbase=735e3  OutputType=Magnitude  PhasorSimulation=off  PSBequivalent=0
  MIC-LTD 409 km : spsDistributedParametersLineLib/Distributed Parameters Line  Phases=3  Length=409  Frequency=60  Resistance="[0.01273  0.3864]"  Inductance="[0.9337e-3  4.1264e-3]"  Capacitance=[12.74e-9 7.751e-9]  x1=[-0.002325 4.99693340991192e-09 0 0;-0.00225 5.00258416334124e-09 0 0;-0.002175 5.00423592753249e-09 0 0;-0.0021 5.00188738209065e-09 0 0;-0.002025 4.99554040440701e-09 0 0;-0.00195 4.98520006815842e-09 0 0;-0.001875 4.97087463925147e-09 0 0;-0.0018 4.95257556921482e-09 0 0;-0.001725 4.9303174860451e-09 0 0;-0.00165 4.90411818251341e-09 0 0;-0.001575 4.87399860194215e-09 0 0;-0.0015 4.83998282146318e-09 0 0;-0.001425 4.80209803277095e-09 138503.934059065 -724390.23852655;-0.00135 4.76037452038589e-09 158927.516108424 -720185.156863685;-0.001275 4.7148456374454e-09 179224.053933078 -715404.370205625;-0.0012 4.66554777904189e-09 199377.322791238 -710051.700240077;-0.001125 4.6125203531291e-09 219371.212468133 -704131.425809512;-0.00105 4.55580574901994e-09 239189.740154274 -697648.279490727;-0.000975 4.49544930350118e-09 258817.063221862 -690607.443811694;-0.0009 4.43149926459188e-09 278237.491889144 -683014.547108726;-0.000825 4.36400675297468e-09 297435.501762586 -674875.659027273;-0.00075 4.2930257211307e-09 316395.746246834 -666197.285669937;-0.000675 4.21861291021073e-09 335103.068812551 -656986.364395596;-0.0006 4.14082780467729e-09 353542.515112307 -647250.258273787;-0.000525 4.05973258475358e-09 371699.344934864 -636996.750198774;-0.00045 3.97539207671761e-09 389559.043988272 -626234.036668029;-0.000375 3.88787370108105e-09 407107.335502368 -614970.721230074;-0.0003 3.79724741869431e-09 424330.191641415 -603215.807606936;-0.000225 3.70358567482089e-09 441213.844717733 -590978.692496707;-0.00015 3.60696334122579e-09 457744.798197382 -578269.158061974;-7.5e-05 3.5074576563241e-09 473909.837489083 -565097.364110101]  x2=[-0.002325 1.3405915054669e-08 0 0;-0.00225 1.34982767448585e-08 0 0;-0.002175 1.35798481191488e-08 0 0;-0.0021 1.36505639706313e-08 0 0;-0.002025 1.37103677701362e-08 0 0;-0.00195 1.37592117114214e-08 0 0;-0.001875 1.37970567493875e-08 0 0;-0.0018 1.38238726312902e-08 0 0;-0.001725 1.38396379209237e-08 0 0;-0.00165 1.38443400157569e-08 0 0;-0.001575 1.38379751570069e-08 0 0;-0.0015 1.38205484326445e-08 0 0;-0.001425 1.37920737733266e-08 -189823.746323616 -705777.196573591;-0.00135 1.37525739412601e-08 -169795.146815461 -710861.533020212;-0.001275 1.37020805120064e-08 -149630.815664894 -715377.617633884;-0.0012 1.36406338492402e-08 -129346.871929713 -719321.840325663;-0.001125 1.35682830724837e-08 -108959.530284185 -722691.048144279;-0.00105 1.34850860178407e-08 -88485.088057284 -725482.547796553;-0.000975 1.33911091917638e-08 -67939.9122048577 -727694.107800373;-0.0009 1.32864277178898e-08 -47340.4262261302 -729323.960268511;-0.000825 1.31711252769873e-08 -26703.0970350105 -730370.802321841;-0.00075 1.30452940400633e-08 -6044.42179669201 -730833.797130843;-0.000675 1.29090345946834e-08 14619.085259928 -730712.57458455;-0.0006 1.27624558645634e-08 35270.9060434707 -730007.231586412;-0.000525 1.26056750224974e-08 55894.5318043853 -728718.33197683;-0.00045 1.24388173966917e-08 76473.4763317904 -726846.906082429;-0.000375 1.22620163705793e-08 96991.2891322993 -724394.449892436;-0.0003 1.20754132761955e-08 117431.568580292 -721362.923862806;-0.000225 1.18791572811987e-08 137777.975029126 -717754.751349063;-0.00015 1.16734052696285e-08 158014.243872794 -713572.816669108;-7.5e-05 1.14583217164948e-08 178124.19854761 -708820.462797537]  x3=[-0.002325 3.60533395081142e-12 0 0;-0.00225 4.083779441553e-12 0 0;-0.002175 4.55896042149294e-12 0 0;-0.0021 5.03049703822635e-12 0 0;-0.002025 5.49801235259661e-12 0 0;-0.00195 5.9611326400146e-12 0 0;-0.001875 6.41948768920856e-12 0 0;-0.0018 6.87271109816521e-12 0 0;-0.001725 7.320440567026e-12 0 0;-0.00165 7.76231818770401e-12 0 0;-0.001575 8.19799072999021e-12 0 0;-0.0015 8.62710992392033e-12 0 0;-0.001425 9.04933273817647e-12 -163.959464484115 -404.071950169561;-0.00135 9.46432165430115e-12 -152.470711052539 -408.545860687239;-0.001275 9.87174493650435e-12 -140.860074867428 -412.693185894845;-0.0012 1.02712768968481e-11 -129.136837293699 -416.510610484064;-0.001125 1.06625981555963e-11 -117.310369708097 -419.995082864088;-0.00105 1.10453958965221e-11 -105.39012600786 -423.14381760101;-0.000975 1.14193641169685e-11 -93.3856350534147 -425.95429764446;-0.0009 1.17842038724619e-11 -81.306493051156 -428.424276339693;-0.000825 1.2139623515684e-11 -69.1623558823833 -430.55177922353;-0.00075 1.24853389296102e-11 -56.9629313845378 -432.33510560272;-0.000675 1.28210737546281e-11 -44.7179715909055 -433.772829913439;-0.0006 1.31465596094555e-11 -32.4372649349914 -434.863802860873;-0.000525 1.34615363056803e-11 -20.130628425795 -435.607152337939;-0.00045 1.37657520557508e-11 -7.80789980024402 -436.002284122439;-0.000375 1.40589636742509e-11 4.52107034094241 -436.04888235207;-0.0003 1.43409367722992e-11 16.846426407673 -435.74690977692;-0.000225 1.46114459449154e-11 29.1583156988923 -435.096607789246;-0.00015 1.48702749512059e-11 41.446896278679 -434.098496230507;-7.5e-05 1.51172168872232e-11 53.7023448437394 -432.753372975811]  x4=[-0.002325 1.65100914587502e-11 0 0;-0.00225 1.6415084953531e-11 0 0;-0.002175 1.63069564805593e-11 0 0;-0.0021 1.61857924760817e-11 0 0;-0.002025 1.60516897967498e-11 0 0;-0.00195 1.59047556421934e-11 0 0;-0.001875 1.57451074693275e-11 0 0;-0.0018 1.55728728984589e-11 0 0;-0.001725 1.53881896112682e-11 0 0;-0.00165 1.51912052407494e-11 0 0;-0.001575 1.49820772531945e-11 0 0;-0.0015 1.47609728223167e-11 0 0;-0.001425 1.45280686956153e-11 -1447.81766818186 -4750.17763764045;-0.00135 1.42835510530856e-11 -1312.94851541785 -4789.2095920443;-0.001275 1.40276153583896e-11 -1177.02981169941 -4824.41312557762;-0.0012 1.37604662026059e-11 -1040.17020835866 -4855.76009707436;-0.001125 1.34823171406819e-11 -902.479108868481 -4883.22544824512;-0.00105 1.31933905207221e-11 -764.066581387066 -4906.7872237084;-0.000975 1.28939173062457e-11 -625.043270771102 -4926.42658854142;-0.0009 1.25841368915582e-11 -485.520310127966 -4942.12784333641;-0.000825 1.22642969103834e-11 -345.609231977624 -4953.87843675052;-0.00075 1.19346530379084e-11 -205.421879095238 -4961.66897553918;-0.000675 1.15954687864013e-11 -65.0703151057626 -4965.49323206488;-0.0006 1.12470152945629e-11 75.3332650979987 -4965.34814927546;-0.000525 1.08895711107831e-11 215.676625042278 -4961.23384314788;-0.00045 1.05234219704734e-11 355.847576392462 -4953.15360259551;-0.000375 1.01488605676543e-11 495.734068634728 -4941.11388683902;-0.0003 9.76618632098015e-12 635.224278647514 -4925.12432024297;-0.000225 9.37570513438868e-12 774.206700091206 -4905.19768462224;-0.00015 8.97772915256588e-12 912.570232544604 -4881.34990902447;-7.5e-05 8.57257651142238e-12 1050.2042703169 -4853.60005699658]  x5=0.00231306500901259  V1=ones(3,3)  V2=ones(3,3)  I1=ones(3,3)  I2=ones(3,3)  nHarmo=1  Measurements=None  Decoupling=on  VsMag0=[602176.30241456 602177.10748301 602176.165720832]  VrMag0=[596743.7373363 596743.911083318 596743.706580261]  VsAngle0=[11.6043495452618 -108.395709698239 131.604253585471]  VrAngle0=[-14.2738568821649 -134.273869923457 105.726122150019]  IsMag0=[359.486265157327 359.489496854333 359.491918798002]  IrMag0=[4093.84062560503 4093.84102057843 4093.83505039124]  IsAngle0=[-21.306474748612 -141.305731641622 98.6934507450219]  IrAngle0=[-16.1707432095096 -136.170836500558 103.829205357663]
      settings: AttributesFormatString=\n  LibrarySourceBlock=sps_lib/Power Grid Elements/Distributed Parameters Line
  MIC-MAN 60 km : spsDistributedParametersLineLib/Distributed Parameters Line  Phases=3  Length=60  Frequency=60  Resistance="[0.01273  0.3864]"  Inductance="[0.9337e-3  4.1264e-3]"  Capacitance=[12.74e-9 7.751e-9]  x1=[-0.000375 4.13920973953947e-09 367056.472396749 -647795.562767757;-0.0003 4.06279141556716e-09 385223.31391593 -637159.785534167;-0.000225 3.98312535830005e-09 403082.213812081 -626014.672516893;-0.00015 3.90027525156537e-09 420618.895953875 -614369.132948754;-7.5e-05 3.8143073244708e-09 437819.341785928 -602232.476095899]  x2=[-0.000375 8.18431025456971e-10 381674.193271352 -619636.360456955;-0.0003 7.83998581777177e-10 399039.114850708 -608598.586308945;-0.000225 7.48939421626691e-10 416085.050667155 -597074.30776291;-0.00015 7.13281570761714e-10 432798.374460414 -585072.737150793;-7.5e-05 6.77053533522643e-10 449165.725855166 -572603.46834451]  x3=[-0.000375 -1.90049861303933e-11 2615.73591803642 -3083.53120523781;-0.0003 -1.98470969372403e-11 2701.86358792147 -3008.35057124389;-0.000225 -2.06733422784665e-11 2785.83142939423 -2930.76510783263;-0.00015 -2.1483061666188e-11 2867.57231984698 -2850.83683563638;-7.5e-05 -2.22756078231153e-11 2947.02091686258 -2768.62964809299]  x4=[-0.000375 2.6773698317838e-11 -38.3285845654161 -1696.07516225623;-0.0003 2.76635320753654e-11 9.63578970439525 -1696.48092157445;-0.000225 2.8531252028618e-11 57.5924612713494 -1695.53054000099;-0.00015 2.93761645355417e-11 105.503094305957 -1693.22477725634;-7.5e-05 3.01975941860061e-11 153.329389781229 -1689.56547653197]  x5=0.000339324940197445  V1=ones(3,3)  V2=ones(3,3)  I1=ones(3,3)  I2=ones(3,3)  nHarmo=1  Measurements=None  Decoupling=on  VsMag0=[607930.231676096 607930.976808471 607930.152146782]  VrMag0=[594207.380493459 594208.101305642 594207.286862208]  VsAngle0=[7.63692875075284 -112.363120449628 127.636843332424]  VrAngle0=[9.73160889880125 -110.268441654035 129.731523430557]  IsMag0=[3306.19691878131 3306.2003520722 3306.19654855212]  IrMag0=[1387.14843174281 1387.1508825633 1387.14865267738]  IsAngle0=[18.407695376132 -101.592346383788 138.407622969122]  IrAngle0=[-23.1945765462459 -143.194624454327 96.8053118315562]
      settings: AttributesFormatString=\n  LibrarySourceBlock=sps_lib/Power Grid Elements/Distributed Parameters Line
  Regulateurs6 : Subsystem
  Regulateurs7 : Subsystem
  "MIC7a " : PMIOPort  Side=Left
  MIC7b : PMIOPort  Port=2  Side=Left
  MIC7c : PMIOPort  Port=3  Side=Left
  QUE7a : PMIOPort  Port=4  Side=Left
  QUE7b : PMIOPort  Port=5  Side=Left
  QUE7c : PMIOPort  Port=6  Side=Left
  wires:
  Regulateurs6/1(Pm) -> "B_6 CHU-5600 MVA "/1
  Regulateurs6/2(Vf) -> "B_6 CHU-5600 MVA "/2
  "B_6 CHU-5600 MVA "/1 -> Regulateurs6/1(m)
  Regulateurs7/1(Pm) -> B_7 MAN 5000 MVA/1
  Regulateurs7/2(Vf) -> B_7 MAN 5000 MVA/2
  B_7 MAN 5000 MVA/1 -> Regulateurs7/1(m)
  connections:
  "Cs PER "/RConn3 -- MIC-LTD 409 km/LConn3
  "Cs PER "/RConn2 -- MIC-LTD 409 km/LConn2
  "Cs PER "/RConn1 -- MIC-LTD 409 km/LConn1
  Cs BER/RConn3 -- MAN-LEV 3*379km/LConn3
  Cs BER/RConn2 -- MAN-LEV 3*379km/LConn2
  Cs BER/RConn1 -- MAN-LEV 3*379km/LConn1
  Cs ARNS2/RConn3 -- ARN-MAN 2*169km/LConn3
  Cs ARNS2/RConn2 -- ARN-MAN 2*169km/LConn2
  Cs ARNS2/RConn1 -- ARN-MAN 2*169km/LConn1
  CHU-ARN 3*450km/RConn3 -- "Cs MTG+ARNN "/LConn3
  CHU-ARN 3*450km/RConn2 -- "Cs MTG+ARNN "/LConn2
  CHU-ARN 3*450km/RConn1 -- "Cs MTG+ARNN "/LConn1
  Load Flow Bus2/LConn1 -- 5600 MVA 13.8 kV/735 kV1/RConn3 -- CHU-ARN 3*450km/LConn3 -- CHU 330 Mvar/LConn3
  5600 MVA 13.8 kV/735 kV1/RConn2 -- CHU-ARN 3*450km/LConn2 -- CHU 330 Mvar/LConn2
  5600 MVA 13.8 kV/735 kV1/RConn1 -- CHU-ARN 3*450km/LConn1 -- CHU 330 Mvar/LConn1
  "B_6 CHU-5600 MVA "/RConn3 -- Load Flow Bus1/LConn1 -- 5600 MVA 13.8 kV/735 kV1/LConn3 -- 280 MW/LConn3
  5600 MVA 13.8 kV/735 kV1/LConn2 -- "B_6 CHU-5600 MVA "/RConn2 -- 280 MW/LConn2
  5600 MVA 13.8 kV/735 kV1/LConn1 -- "B_6 CHU-5600 MVA "/RConn1 -- 280 MW/LConn1
  "Cs ARNS1 "/RConn1 -- ARN-MIC 180km/LConn1
  "Cs ARNS1 "/RConn2 -- ARN-MIC 180km/LConn2
  "Cs ARNS1 "/RConn3 -- ARN-MIC 180km/LConn3
  "Cs PER "/LConn3 -- Load Flow Bus6/LConn1 -- MIC7c/RConn1 -- MIC-MAN 60 km/LConn3 -- ARN-MIC 180km/RConn3
  "Cs PER "/LConn2 -- MIC7b/RConn1 -- ARN-MIC 180km/RConn2 -- MIC-MAN 60 km/LConn2
  "Cs PER "/LConn1 -- "MIC7a "/RConn1 -- ARN-MIC 180km/RConn1 -- MIC-MAN 60 km/LConn1
  ARN-MAN 2*169km/RConn1 -- MAN7/LConn1
  ARN-MAN 2*169km/RConn2 -- MAN7/LConn2
  ARN-MAN 2*169km/RConn3 -- MAN7/LConn3
  Cs BER/LConn1 -- 5000 MVA 13.8 kV/735 kV2/RConn1 -- MIC-MAN 60 km/RConn1 -- MAN-MIC 1650 Mvar/LConn1 -- MAN7/RConn1
  Cs BER/LConn2 -- 5000 MVA 13.8 kV/735 kV2/RConn2 -- MIC-MAN 60 km/RConn2 -- MAN-MIC 1650 Mvar/LConn2 -- MAN7/RConn2
  Cs BER/LConn3 -- Load Flow Bus5/LConn1 -- 5000 MVA 13.8 kV/735 kV2/RConn3 -- MIC-MAN 60 km/RConn3 -- MAN-MIC 1650 Mvar/LConn3 -- MAN7/RConn3
  B_7 MAN 5000 MVA/RConn1 -- 5000 MVA 13.8 kV/735 kV2/LConn1 -- 250 MW/LConn1
  B_7 MAN 5000 MVA/RConn2 -- 5000 MVA 13.8 kV/735 kV2/LConn2 -- 250 MW/LConn2
  B_7 MAN 5000 MVA/RConn3 -- 5000 MVA 13.8 kV/735 kV2/LConn3 -- Load Flow Bus3/LConn1 -- 250 MW/LConn3
  MIC-LTD 409 km/RConn2 -- MAN-LEV 3*379km/RConn2 -- QUE7b/RConn1
  Cs ARNS2/LConn1 -- ARN 990 Mvar/LConn1 -- "Cs MTG+ARNN "/RConn1 -- "Cs ARNS1 "/LConn1
  Cs ARNS2/LConn2 -- ARN 990 Mvar/LConn2 -- "Cs MTG+ARNN "/RConn2 -- "Cs ARNS1 "/LConn2
  Cs ARNS2/LConn3 -- Load Flow Bus4/LConn1 -- "Cs ARNS1 "/LConn3 -- ARN 990 Mvar/LConn3 -- "Cs MTG+ARNN "/RConn3
  MIC-LTD 409 km/RConn1 -- QUE7a/RConn1 -- MAN-LEV 3*379km/RConn1
  MIC-LTD 409 km/RConn3 -- QUE7c/RConn1 -- MAN-LEV 3*379km/RConn3
